simulink model "sysgenFloatingPointFIR"  (Simulink 7.5)
settings: Solver=VariableStepDiscrete  SolverMode=SingleTasking  StartTime=0.0  StopTime=30000  RelTol=1e-3
PreLoadFcn:
  | sysgenFloatingPointFIR_PreLoadFcn
undefined symbols (not defined in the file or in its folder): get, One, sided
libraries: xbsIndex_r4 x18, sysgenFloatingPointFIR_Lib x5, dspsnks4 x2, simulink x1, xbsCopyrightNotice_r4 x1
settings Model: Creator=jayeshs  LastModifiedBy=arvinds
settings OptimizationCC: InlineParams=on

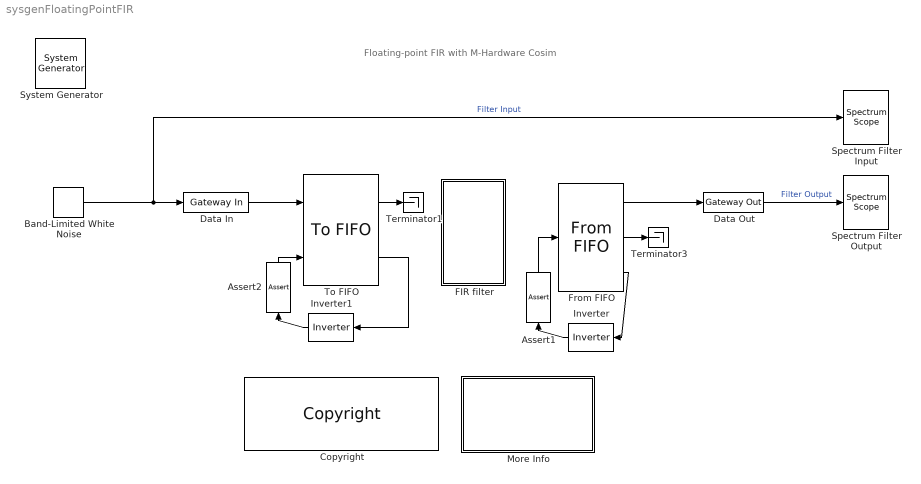
== system sysgenFloatingPointFIR ==
  note: Floating-point FIR with M-Hardware Cosim
  " System Generator" : xbsIndex_r4/ System Generator  Tag=genX  SystemSampleTime=-1  xilinxfamily=spartan6  part=xc6slx45t  speed=-3  package=fgg484  synthesis_tool=XST  clock_wrapper=Clock Enables  directory=./netlist  proj_type=Project Navigator  Synth_file=XST Defaults  Impl_file=ISE Defaults  testbench=on  simulink_period=1  sysclk_period=10  dcm_input_clock_period=10  incr_netlist=off  trim_vbits=Everywhere in SubSystem  dbl_ovrd=According to Block Masks  core_generation=According to Block Masks  run_coregen=off  deprecated_control=off  eval_field=0  block_type=sysgen
      settings: block_version=13.2
  Assert1 : xbsIndex_r4/Assert  assert_type=off  type_source=Explicitly  gui_display_data_type=Fixed-point  arith_type=Unsigned  n_bits=8  bin_pt=2  preci_type=Single  exp_width=8  frac_width=24  assert_rate=on  rate_source=Explicitly  period=1  output_port=on  block_type=assert
      settings: infoedit=Asserts a user-defined sample rate and/or type on a signal.  block_version=VER_STRING_GOES_HERE
  Assert2 : xbsIndex_r4/Assert  assert_type=off  type_source=Explicitly  gui_display_data_type=Fixed-point  arith_type=Unsigned  n_bits=8  bin_pt=2  preci_type=Single  exp_width=8  frac_width=24  assert_rate=on  rate_source=Explicitly  period=1  output_port=on  block_type=assert
      settings: infoedit=Asserts a user-defined sample rate and/or type on a signal.  block_version=VER_STRING_GOES_HERE
  Band-Limited White Noise : simulink/Sources/Band-Limited White Noise  SystemSampleTime=-1  Cov=[1]  Ts=1  seed=[23341]
  Copyright : xbsCopyrightNotice_r4/Copyright  copyrighttext="Copyright (c) 2011  by  Xilinx, Inc. All rights reserved.<br><br>This file contains proprietary, confidential information of Xilinx, Inc., is distributed under license from Xilinx, Inc., and may be used, copied and/or disclosed only pursuant to the terms of a valid license agreement with Xilinx, Inc. Xilinx hereby grants you a license to use this file solely for design, simulation, implementation and creation of design files limited to Xilinx devices or technologies. Use with non-Xilinx devices or technologies is expressly prohibited and immediately terminates your license unless covered by a separate agreement.<br><br>Xilinx is providing this design, code, or information \"as-is\" solely for use in developing programs and solutions for Xilinx devices, with no obligation on the part of Xilinx to provide support. By providing this design, code, or information as one possible implementation of this feature, application or standard, Xilinx is making no representation that this implementation is free from any claims of infringement. You are responsible for obtaining any rights you may require for your implementation. Xilinx expressly disclaims any warranty whatsoever with respect to the adequacy of the implementation, including but not limited to any warranties or representations that this implementation is free from claims of infringement, implied warranties of merchantability or fitness for a particular purpose.<br><br>Xilinx products are not intended for use in life support appliances, devices, or systems. Use in such applications is expressly prohibited.<br><br>Any modifications that are made to the Source Code are done at the user's sole risk and will be unsupported.<br><br>This copyright and support notice must be retained as part of this text at all times. (c) Copyright 1995-2011 Xilinx, Inc. All rights reserved."  block_type=copyright
      settings: block_version=10.1.00
      settings: infoedit=|
      | Copyright(C) 2008 by  Xilinx, Inc. All rights reserved.<br>
      | <br>
      | This file contains proprietary, confidential information of Xilinx, Inc., is distributed under license
      | from Xilinx, Inc., and may be used, copied and/or disclosed only pursuant to the terms of a valid license
      | agreement with Xilinx, Inc. Xilinx hereby grants you a license to use this file solely for design,
      | simulation, implementation and creation of design files limited to Xilinx devices or technologies. Use
      | with non-Xilinx devices or technologies is expressly prohibited and immediately terminates your license
      | unless covered by a separate agreement.<br>
      | <br>
      | Xilinx is providing this design, code, or information "as-is" solely for use in developing programs and
      | solutions for Xilinx devices, with no obligation on the part of Xilinx to provide support. By providing
      | this design, code, or information as one possible implementation of this feature, application or standard,
      | Xilinx is making no representation that this implementation is free from any claims of infringement. You
      | are responsible for obtaining any rights you may require for your implementation. Xilinx expressly disclaims
      | any warranty whatsoever with respect to the adequacy of the implementation, including but not limited to any
      | warranties or representations that this implementation is free from claims of infringement, implied warranties
      | of merchantability or fitness for a particular purpose.<br>
      | <br>
      | Xilinx products are not intended for use in life support appliances, devices, or systems. Use in such
      | applications is expressly prohibited.<br>
      | <br>
      | Any modifications that are made to the Source Code are done at the user's sole risk and will be unsupported.<br>
      | <br>
      | This copyright and support notice must be retained as part of this text at all times.
      | (c) Copyright 1995-2008 Xilinx, Inc. All rights reserved.
  Data In : xbsIndex_r4/Gateway In  gui_display_data_type=Floating-point  arith_type=Floating-point  n_bits=40  bin_pt=32  preci_type=Single  exp_width=6  frac_width=15  quantization="Round  (unbiased: +/- Inf)"  overflow=Saturate  period=1  dbl_ovrd=off  timing_constraint=None  locs_specified=off  LOCs={}  hdl_port=on  block_type=gatewayin
      settings: infoedit="Gateway in block.  Converts inputs of type Simulink integer, double and fixed point to  Xilinx fixed point or floating-point data type.<br><br>Hardware notes:  In hardware these blocks become top level input ports."  block_version=13.2
  Data Out : xbsIndex_r4/Gateway Out  hdl_port=on  timing_constraint=None  locs_specified=off  LOCs={}  block_type=gatewayout
      settings: infoedit="Gateway out block.  Converts Xilinx fixed point inputs into ouputs of type Simulink integer, double, or fixed point.<br><br>Hardware notes:  In hardware these blocks become top level output ports or are discarded, depending on how they are configured."  block_version=13.2
  FIR filter : Subsystem
  From FIFO : xbsIndex_r4/From FIFO  shared_memory_name='VA'  ownership=Owned elsewhere  performance_options=Standard_FIFO  depth=4K  percent_nbits=8  has_arst=off  use_percent_full_port=on  gui_display_data_type=Floating-point  arith_type=Floating-point  n_bits=32  bin_pt=29  preci_type=Single  dbl_ovrd=off  mem_type=Block RAM  block_type=fromfifo
      settings: AttributesFormatString=<< %<shared_memory_name> >>  infoedit=First-in-first-out (FIFO) block that reads FIFO data from shared memory storage.  block_version=VER_STRING_GOES_HERE
  Inverter : xbsIndex_r4/Inverter  en=off  latency=0  dbl_ovrd=off  block_type=inv
      settings: block_version=VER_STRING_GOES_HERE
  Inverter1 : xbsIndex_r4/Inverter  en=off  latency=0  dbl_ovrd=off  block_type=inv
      settings: block_version=VER_STRING_GOES_HERE
  More Info : Subsystem
      mask Display: disp('Double click\n for\n more information.')
  Spectrum Filter Input : dspsnks4/Spectrum Scope  DialogController=dspdialog.SpectrumScope  DialogControllerArgs=DataTag2  SystemSampleTime=-1  ScopeProperties=on  Domain=Frequency  HorizSpan=1  UseBuffer=on  BufferSize=1024  Overlap=64  inpFftLenInherit=off  FFTlength=128  numAvg=20  DisplayProperties=off  AxisGrid=on  Memory=off  FrameNumber=on  AxisLegend=off  AxisZoom=off  OpenScopeAtSimStart=on  OpenScopeImmediately=off  FigPos=get(0,'defaultfigureposition')  AxisProperties=off  XUnits=Hertz  XRange=One-sided ([0...Fs/2])  XDisplay=0  InheritXIncr=off  XIncr=1.0  XLabel=Samples  XLimit=Auto  YUnits=dBW/Hertz  XMax=1  XMin=0  YLabel=Magnitude-squared, dB  LineProperties=off  wintypeSpecScope=Hann  RsSpecScope=50  betaSpecScope=5  winsampSpecScope=Periodic  XAxisParamsVer=6.9
      settings: YMin=-10  YMax=10
  Spectrum Filter Output : dspsnks4/Spectrum Scope  DialogController=dspdialog.SpectrumScope  DialogControllerArgs=DataTag3  SystemSampleTime=-1  ScopeProperties=on  Domain=Frequency  HorizSpan=1  UseBuffer=on  BufferSize=1024  Overlap=64  inpFftLenInherit=off  FFTlength=128  numAvg=20  DisplayProperties=off  AxisGrid=on  Memory=off  FrameNumber=on  AxisLegend=off  AxisZoom=off  OpenScopeAtSimStart=on  OpenScopeImmediately=off  FigPos=get(0,'defaultfigureposition')  AxisProperties=off  XUnits=Hertz  XRange=One-sided ([0...Fs/2])  XDisplay=0  InheritXIncr=off  XIncr=1.0  XLabel=Samples  XLimit=Auto  YUnits=dBW/Hertz  XMax=1  XMin=0  YLabel=Magnitude-squared, dB  LineProperties=off  wintypeSpecScope=Hann  RsSpecScope=50  betaSpecScope=5  winsampSpecScope=Periodic  XAxisParamsVer=6.9
      settings: YMin=-10  YMax=10
  Terminator1 : Terminator
  Terminator3 : Terminator
  To FIFO : xbsIndex_r4/To FIFO  shared_memory_name='CA'  ownership=Owned elsewhere  performance_options=Standard_FIFO  depth=4K  percent_nbits=1  has_arst=off  use_percent_full_port=on  explicit_data_type=off  gui_display_data_type=Fixed-point  arith_type="Signed  (2's comp)"  n_bits=32  bin_pt=11  preci_type=Single  dbl_ovrd=off  mem_type=Block RAM  block_type=tofifo
      settings: AttributesFormatString=<< %<shared_memory_name> >>  infoedit=First-in-first-out (FIFO) block that writes FIFO data to shared memory storage.  block_version=VER_STRING_GOES_HERE
  wires:
  Band-Limited White Noise/1 -> Data In/1, Spectrum Filter Input/1  "Filter Input"
  From FIFO/2 -> Terminator3/1
  From FIFO/3 -> Inverter/1
  Inverter/1 -> Assert1/1
  Assert1/1 -> From FIFO/1
  From FIFO/1 -> Data Out/1
  To FIFO/1 -> Terminator1/1
  To FIFO/2 -> Inverter1/1
  Assert2/1 -> To FIFO/2
  Inverter1/1 -> Assert2/1
  Data In/1 -> To FIFO/1
  Data Out/1 -> Spectrum Filter Output/1  "Filter Output"

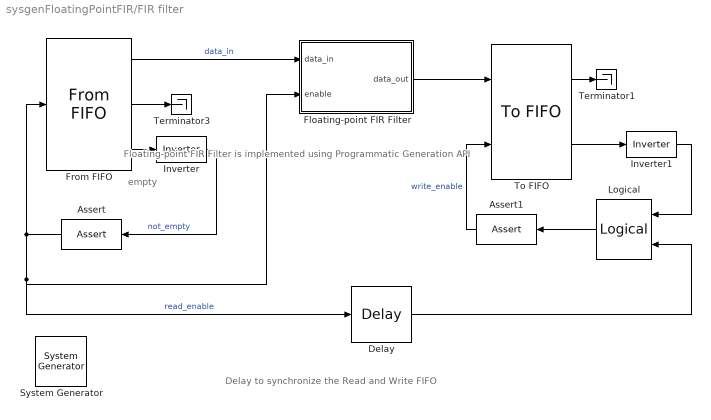
== system sysgenFloatingPointFIR/FIR filter ==
  note: empty
  note: Floating-point FIR Filter is
      |          implemented using
      | Programmatic Generation API
  note: Delay to synchronize the
      |      Read and Write FIFO
  " System Generator" : xbsIndex_r4/ System Generator  Tag=genX  SystemSampleTime=-1  xilinxfamily=spartan6  part=xc6slx45t  speed=-3  package=fgg484  synthesis_tool=XST  clock_wrapper=Clock Enables  directory=./netlist  proj_type=Project Navigator  Synth_file=XST Defaults  Impl_file=ISE Defaults  testbench=off  simulink_period=1  sysclk_period=20  dcm_input_clock_period=100  incr_netlist=off  trim_vbits=Everywhere in SubSystem  dbl_ovrd=According to Block Masks  core_generation=According to Block Masks  run_coregen=off  deprecated_control=off  eval_field=0  block_type=sysgen
      settings: block_version=8.2.02
  Assert : xbsIndex_r4/Assert  assert_type=off  type_source=Explicitly  gui_display_data_type=Fixed-point  arith_type=Unsigned  n_bits=8  bin_pt=2  preci_type=Single  exp_width=8  frac_width=24  assert_rate=on  rate_source=Explicitly  period=1  output_port=on  block_type=assert
      settings: infoedit=Asserts a user-defined sample rate and/or type on a signal.  block_version=VER_STRING_GOES_HERE
  Assert1 : xbsIndex_r4/Assert  assert_type=off  type_source=Explicitly  gui_display_data_type=Fixed-point  arith_type=Unsigned  n_bits=8  bin_pt=2  preci_type=Single  exp_width=8  frac_width=24  assert_rate=on  rate_source=Explicitly  period=1  output_port=on  block_type=assert
      settings: infoedit=Asserts a user-defined sample rate and/or type on a signal.  block_version=VER_STRING_GOES_HERE
  Delay : xbsIndex_r4/Delay  rst=off  infoeditControl=Selection of Reset will increase slice count due to use of real FFs and instead of SRLs  en=off  latency=3  dbl_ovrd=off  reg_retiming=off  block_type=delay
  Floating-point FIR Filter : Subsystem  mask{filter_coefficients=fir1(4,0.02)}
      mask prompts: filter_coefficients "Filter Coefficients"
      mask init:
      | config.source = str2func('sysgenFloatingPointFIRGenerator'); 
      | config.toplevel = gcb; 
      | xBlock(config, {filter_coefficients});
  From FIFO : xbsIndex_r4/From FIFO  shared_memory_name='CA'  ownership=Locally owned  performance_options=Standard_FIFO  depth=4K  percent_nbits=1  has_arst=off  use_percent_full_port=on  gui_display_data_type=Floating-point  arith_type=Floating-point  n_bits=32  bin_pt=24  preci_type=Single  dbl_ovrd=off  mem_type=Block RAM  block_type=fromfifo
      settings: AttributesFormatString=<< %<shared_memory_name> >>  infoedit=First-in-first-out (FIFO) block that reads FIFO data from shared memory storage.  block_version=VER_STRING_GOES_HERE
  Inverter : xbsIndex_r4/Inverter  en=off  latency=0  dbl_ovrd=off  block_type=inv
      settings: block_version=VER_STRING_GOES_HERE
  Inverter1 : xbsIndex_r4/Inverter  en=off  latency=0  dbl_ovrd=off  block_type=inv
      settings: block_version=VER_STRING_GOES_HERE
  Logical : xbsIndex_r4/Logical  logical_function=AND  inputs=2  en=off  latency=0  precision=Full  arith_type=Unsigned  n_bits=16  bin_pt=0  align_bp=on  dbl_ovrd=off  block_type=logical
  Terminator1 : Terminator
  Terminator3 : Terminator
  To FIFO : xbsIndex_r4/To FIFO  shared_memory_name='VA'  ownership=Locally owned  performance_options=Standard_FIFO  depth=4K  percent_nbits=8  has_arst=off  use_percent_full_port=on  explicit_data_type=on  gui_display_data_type=Floating-point  arith_type=Floating-point  n_bits=32  bin_pt=24  preci_type=Single  dbl_ovrd=off  mem_type=Block RAM  block_type=tofifo
      settings: AttributesFormatString=<< %<shared_memory_name> >>  infoedit=First-in-first-out (FIFO) block that writes FIFO data to shared memory storage.  block_version=VER_STRING_GOES_HERE
  wires:
  Inverter/1 -> Assert/1  "not_empty"
  From FIFO/3 -> Inverter/1
  Assert/1 -> From FIFO/1, Delay/1, Floating-point FIR Filter/2(enable)  "read_enable"
  To FIFO/1 -> Terminator1/1
  To FIFO/2 -> Inverter1/1
  Logical/1 -> Assert1/1
  Assert1/1 -> To FIFO/2  "write_enable"
  From FIFO/1 -> Floating-point FIR Filter/1(data_in)  "data_in"
  Delay/1 -> Logical/2
  Inverter1/1 -> Logical/1
  Floating-point FIR Filter/1(data_out) -> To FIFO/1
  From FIFO/2 -> Terminator3/1

== system sysgenFloatingPointFIR/More Info ==
  note: Sysgen Floating Point FIR using M-Hardware Cosim
  note: This model implements a transposed FIR filter with single precision floating point inputs. The floating
      | point data is communicated to/from the FIR filter using the Shared FIFO.
      |
      | The read enable on the input FIFO is asserted only when the FIFO is not empty. The write enable on the
      | output FIFO is asserted when the FIFO is not full and the delayed read enable signal from the input FIFO is
      | high. The delayed read enable signal is used from the input FIFO for synchronization with the output FIFO,
      | when the subsytem is free-running. This ensures that  the correct samples are read out from the
      | output FIFO.
      |
      | The amount of delay required between the input and the output FIFO is equal to the clock cycles required by
      | the subsystem to produce the first output + 1(1 is added to account for the delay between read enable on
      | the FIFO and when the data sample first appears on the output of the FIFO).
      |
      | The subsystem also contains an enable input. This signal is used for synchronization in the internal circuitry.
      | It ensures that the correct data samples are propagated through the internal circuitry only when there is valid
      | data in the input FIFO.
      |
      | The FIR subsystem takes in the coefficients of the filters and implements a transposed FIR Filter. When the
      | coefficients are given to the block, internally the 'sysgenFloatingPointFIRGenerator.m' script is run. This is
      | used for programmatic generation of Xilinx based simulink blocks and models. Please refer the section on
      | Programmatic Access in the SysGen User Guide for more details on Programmatic Generation API (PGAPI).
      |
      | The files for hardware cosimulation(.hwc, .mdl, .bit) with six tap FIR filter are provided along with this example
      | for SP-605 board. The M-hardware cosimulation script 'mhwcosim_fir_filter.m' will run the simulation on
      | hardware. According to the synchronization circuitry provided, each input sample in the input FIFO will provide
      | a corresponding ouput sample on the output FIFO.  Sifting in zero input can be used to get the remaining data
      | samples in the subsystem out.
      |
      | To generate a Hardware CoSim block for a different board, take the following steps:
      |
      | 1. Go into the FIR filter.
      | 2. Double click on the Xilinx Sysgen token.
      | 3. Under Compilation, select Hardware Co-Simulation, select your board and the connection type.
      | 4. Specify the name of your target directory.
      | 5. Hit Generate.
      | 6. Once the hardware co-sim block is generated for your design, copy the .hwc and the .bit files for the hardware
      |     co-sim block from the target directory to the current directory.
      | 7. Under the Matlab command window, use xlHwcosimConfig('<your block name>.hwc') to configure it as
      |     free-running.
      | 8. Make the changes in sysgenFloatingPointFIR_mhwcosim.m to incorporate your design name.
      | 9. Type sysgenFloatingPointFIR_mhwcosim in the Matlab Console and see your custom FIR filter simulation
      |      run on your FPGA board.

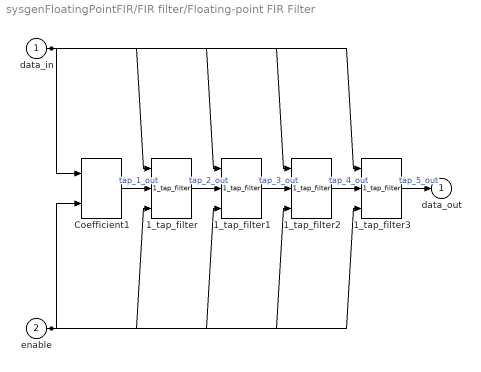
== system sysgenFloatingPointFIR/FIR filter/Floating-point FIR Filter ==
  data_in : Inport
  enable : Inport  Port=2
  1_tap_filter : sysgenFloatingPointFIR_Lib/1_tap_filter  SystemSampleTime=-1  filter_coefficient=0.241034568214606
  1_tap_filter1 : sysgenFloatingPointFIR_Lib/1_tap_filter  SystemSampleTime=-1  filter_coefficient=0.446654140147575
  1_tap_filter2 : sysgenFloatingPointFIR_Lib/1_tap_filter  SystemSampleTime=-1  filter_coefficient=0.241034568214606
  1_tap_filter3 : sysgenFloatingPointFIR_Lib/1_tap_filter  SystemSampleTime=-1  filter_coefficient=0.0356383617116066
  Coefficient1 : sysgenFloatingPointFIR_Lib/Coefficient1  SystemSampleTime=-1  coeff=0.0356383617116066
  data_out : Outport
  wires:
  data_in/1 -> 1_tap_filter3/1, 1_tap_filter2/1, 1_tap_filter1/1, 1_tap_filter/1, Coefficient1/1
  enable/1 -> 1_tap_filter3/3, 1_tap_filter2/3, 1_tap_filter1/3, 1_tap_filter/3, Coefficient1/2
  1_tap_filter3/1 -> data_out/1  "tap_5_out"
  1_tap_filter2/1 -> 1_tap_filter3/2  "tap_4_out"
  1_tap_filter1/1 -> 1_tap_filter2/2  "tap_3_out"
  1_tap_filter/1 -> 1_tap_filter1/2  "tap_2_out"
  Coefficient1/1 -> 1_tap_filter/2  "tap_1_out"
